simulink model "logical_hystersis_prove"  (R2014b)
settings: Solver=FixedStepDiscrete  StartTime=0.0  StopTime=0.03  FixedStep=0.01  RelTol=1e-3
undefined symbols (not defined in the file): sldvsubsys
libraries: sldvlib x16
settings Model: Creator=Natasha  LastModifiedBy=JYOGANAN
settings DebuggingCC: UnderspecifiedInitializationDetection=Classic  MergeDetectMultiDrivingBlocksExec=none

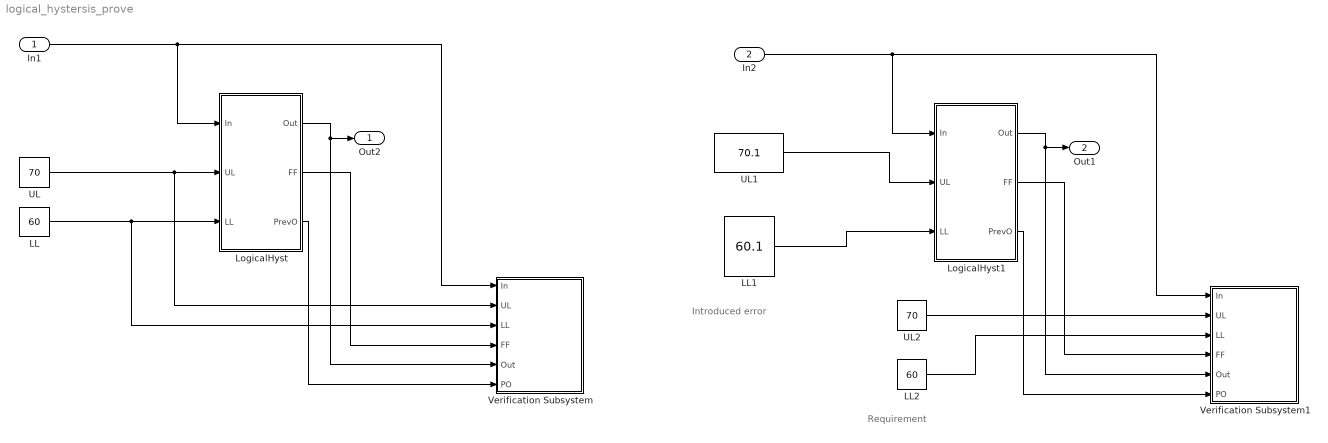
== system logical_hystersis_prove ==
  note: Introduced error
  note: Requirement
  In1 : Inport
  In2 : Inport  Port=2
  LL : Constant  Value=60
  LL1 : Constant  Value=60.1
  LL2 : Constant  Value=60
  LogicalHyst : Subsystem
  LogicalHyst1 : Subsystem
  UL : Constant  Value=70
  UL1 : Constant  Value=70.1
  UL2 : Constant  Value=70
  Verification Subsystem : Subsystem  Tag=VerificationSubsystem  DisableCoverage=on  LoadFcn=sldvsubsys('check')  TreatAsAtomicUnit=on  SimViewingDevice=on  mask(VerificationSubsystem){}
      mask init:
      | sldvsubsys('maskInit');
      settings: CopyFcn=sldvsubsys('copy');  OpenFcn=open_system(gcb,'force');
      settings: PreSaveFcn=|
      | set_param(gcb,'SimViewingDevice','on');
      | sldvsubsys('check');
      mask Help: helpview(fullfile(docroot,'toolbox','sldv','sldv.map'),'verificationsubsystem')
      mask Display: image(imread('sldvicon_versubsys.png','BackGroundColor',[1 1 1]),'center');
  Verification Subsystem1 : Subsystem  Tag=VerificationSubsystem  DisableCoverage=on  LoadFcn=sldvsubsys('check')  TreatAsAtomicUnit=on  SimViewingDevice=on  mask(VerificationSubsystem){}
      mask init:
      | sldvsubsys('maskInit');
      settings: CopyFcn=sldvsubsys('copy');  OpenFcn=open_system(gcb,'force');
      settings: PreSaveFcn=|
      | set_param(gcb,'SimViewingDevice','on');
      | sldvsubsys('check');
      mask Help: helpview(fullfile(docroot,'toolbox','sldv','sldv.map'),'verificationsubsystem')
      mask Display: image(imread('sldvicon_versubsys.png','BackGroundColor',[1 1 1]),'center');
  Out2 : Outport
  Out1 : Outport  Port=2
  wires:
  UL/1 -> Verification Subsystem/2(UL), LogicalHyst/2(UL)
  LL/1 -> Verification Subsystem/3(LL), LogicalHyst/3(LL)
  LogicalHyst/1(Out) -> Verification Subsystem/5(Out), Out2/1
  LogicalHyst/2(FF) -> Verification Subsystem/4(FF)
  In1/1 -> LogicalHyst/1(In), Verification Subsystem/1(In)
  LogicalHyst/3(PrevO) -> Verification Subsystem/6(PO)
  UL1/1 -> LogicalHyst1/2(UL)
  LL1/1 -> LogicalHyst1/3(LL)
  LogicalHyst1/1(Out) -> Verification Subsystem1/5(Out), Out1/1
  LogicalHyst1/2(FF) -> Verification Subsystem1/4(FF)
  In2/1 -> LogicalHyst1/1(In), Verification Subsystem1/1(In)
  LogicalHyst1/3(PrevO) -> Verification Subsystem1/6(PO)
  UL2/1 -> Verification Subsystem1/2(UL)
  LL2/1 -> Verification Subsystem1/3(LL)

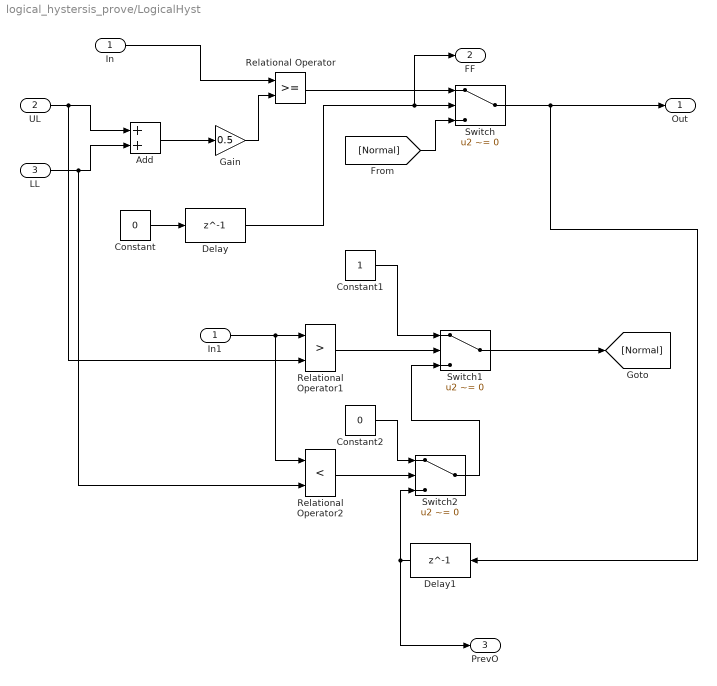
== system logical_hystersis_prove/LogicalHyst ==
  In : Inport
  UL : Inport  Port=2
  LL : Inport  Port=3
  Add : Sum
  Constant : Constant  Value=0
  Constant1 : Constant  OutDataTypeStr=boolean
  Constant2 : Constant  Value=0  OutDataTypeStr=boolean
  Delay : Delay  DelayLength=1  InitialCondition=1
  Delay1 : Delay  DelayLength=1  InitialCondition=0
  Gain : Gain  Gain=0.5
  In1 : InportShadow
  Relational Operator : RelationalOperator  OutDataTypeStr=boolean
  Relational Operator1 : RelationalOperator  Operator=>  OutDataTypeStr=boolean
  Relational Operator2 : RelationalOperator  Operator=<  OutDataTypeStr=boolean
  Switch : Switch  Criteria=u2 ~= 0
  Switch1 : Switch  Criteria=u2 ~= 0
  Switch2 : Switch  Criteria=u2 ~= 0
  Out : Outport
  FF : Outport  Port=2
  PrevO : Outport  Port=3
  wires:
  In/1 -> Relational Operator/1
  Constant/1 -> Delay/1
  Switch/1 -> Delay1/1, Out/1
  UL/1 -> Relational Operator1/2, Add/1
  Delay/1 -> FF/1, Switch/2
  [Normal] -> Switch/3
  Add/1 -> Gain/1
  LL/1 -> Relational Operator2/2, Add/2
  Gain/1 -> Relational Operator/2
  Relational Operator/1 -> Switch/1
  In1/1 -> Relational Operator2/1, Relational Operator1/1
  Relational Operator1/1 -> Switch1/2
  Constant1/1 -> Switch1/1
  Relational Operator2/1 -> Switch2/2
  Constant2/1 -> Switch2/1
  Switch2/1 -> Switch1/3
  Switch1/1 -> [Normal]
  Delay1/1 -> Switch2/3, PrevO/1

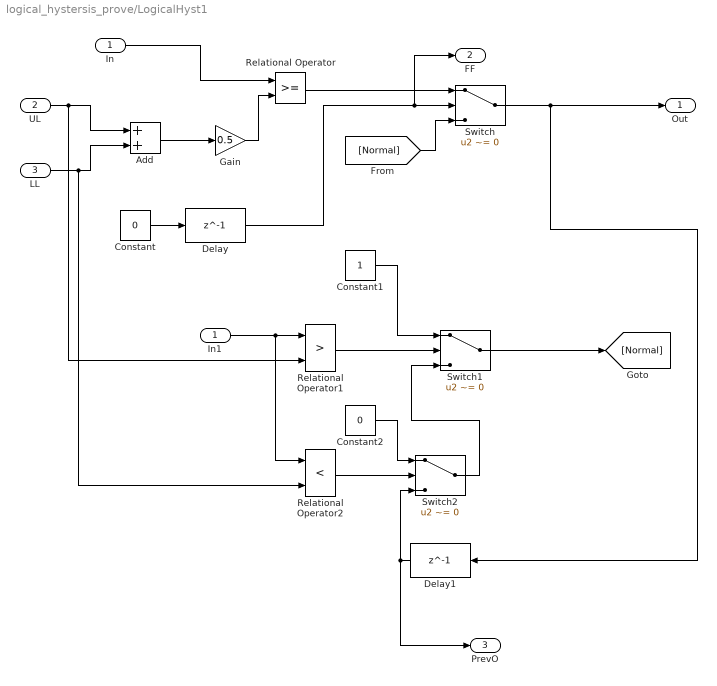
== system logical_hystersis_prove/LogicalHyst1 ==
  In : Inport
  UL : Inport  Port=2
  LL : Inport  Port=3
  Add : Sum
  Constant : Constant  Value=0
  Constant1 : Constant  OutDataTypeStr=boolean
  Constant2 : Constant  Value=0  OutDataTypeStr=boolean
  Delay : Delay  DelayLength=1  InitialCondition=1
  Delay1 : Delay  DelayLength=1  InitialCondition=0
  Gain : Gain  Gain=0.5
  In1 : InportShadow
  Relational Operator : RelationalOperator  OutDataTypeStr=boolean
  Relational Operator1 : RelationalOperator  Operator=>  OutDataTypeStr=boolean
  Relational Operator2 : RelationalOperator  Operator=<  OutDataTypeStr=boolean
  Switch : Switch  Criteria=u2 ~= 0
  Switch1 : Switch  Criteria=u2 ~= 0
  Switch2 : Switch  Criteria=u2 ~= 0
  Out : Outport
  FF : Outport  Port=2
  PrevO : Outport  Port=3
  wires:
  In/1 -> Relational Operator/1
  Constant/1 -> Delay/1
  Switch/1 -> Delay1/1, Out/1
  UL/1 -> Relational Operator1/2, Add/1
  Delay/1 -> FF/1, Switch/2
  [Normal] -> Switch/3
  Add/1 -> Gain/1
  LL/1 -> Relational Operator2/2, Add/2
  Gain/1 -> Relational Operator/2
  Relational Operator/1 -> Switch/1
  In1/1 -> Relational Operator2/1, Relational Operator1/1
  Relational Operator1/1 -> Switch1/2
  Constant1/1 -> Switch1/1
  Relational Operator2/1 -> Switch2/2
  Constant2/1 -> Switch2/1
  Switch2/1 -> Switch1/3
  Switch1/1 -> [Normal]
  Delay1/1 -> Switch2/3, PrevO/1

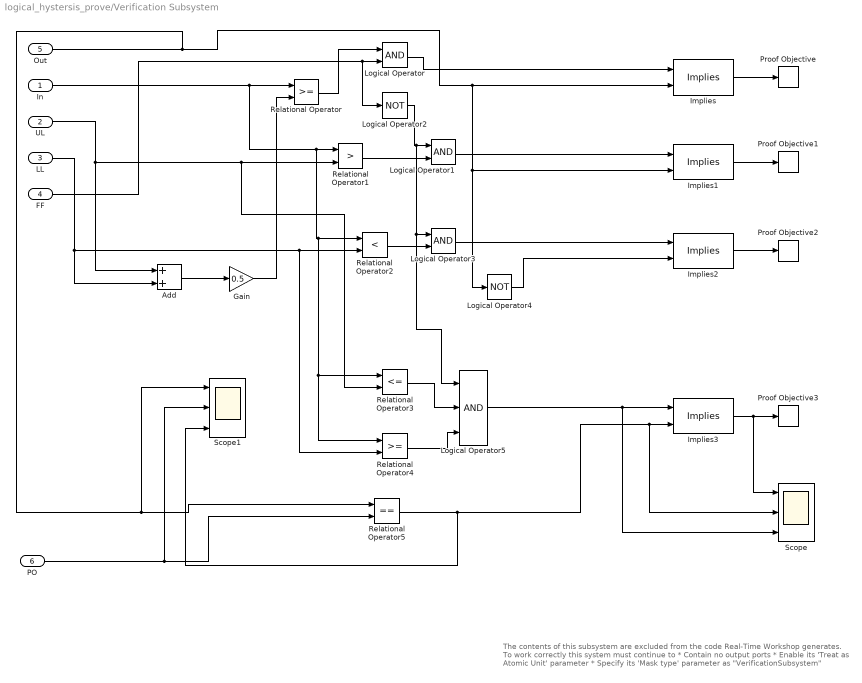
== system logical_hystersis_prove/Verification Subsystem ==
  note: The contents of this subsystem are excluded from the code Real-Time
      | Workshop generates.
      |
      | To work correctly this system must continue to
      | * Contain no output ports
      | * Enable its 'Treat as Atomic Unit' parameter
      | * Specify its 'Mask type' parameter as "VerificationSubsystem"
  In : Inport
  UL : Inport  Port=2
  LL : Inport  Port=3
  FF : Inport  Port=4
  Out : Inport  Port=5
  PO : Inport  Port=6
  Add : Sum
  Gain : Gain  Gain=0.5
  Implies{,1..3} (4 alike) : sldvlib/Verification Utilities/Implies
  Logical Operator : Logic  AllPortsSameDT=off  OutDataTypeStr=boolean
  Logical Operator1 : Logic  AllPortsSameDT=off  OutDataTypeStr=boolean
  Logical Operator2 : Logic  Operator=NOT  AllPortsSameDT=off  OutDataTypeStr=boolean
  Logical Operator3 : Logic  AllPortsSameDT=off  OutDataTypeStr=boolean
  Logical Operator4 : Logic  Operator=NOT  AllPortsSameDT=off  OutDataTypeStr=boolean
  Logical Operator5 : Logic  Inputs=3  AllPortsSameDT=off  OutDataTypeStr=boolean
  Proof Objective{,1..3} (4 alike) : sldvlib/Objectives and Constraints/Proof Objective  enabled=on  customAVTBlockType=Proof Objective  intervals=true  dispValues=on  outEnabled=off  enableStopSim=off
      settings: AttributesFormatString=%<intervals>
  Relational Operator : RelationalOperator  OutDataTypeStr=boolean
  Relational Operator1 : RelationalOperator  Operator=>  OutDataTypeStr=boolean
  Relational Operator2 : RelationalOperator  Operator=<  OutDataTypeStr=boolean
  Relational Operator3 : RelationalOperator  Operator=<=  OutDataTypeStr=boolean
  Relational Operator4 : RelationalOperator  OutDataTypeStr=boolean
  Relational Operator5 : RelationalOperator  Operator===  OutDataTypeStr=boolean
  Scope : Scope  NumInputPorts=3
      settings: YMin=-5~-5~-5  YMax=5~5~5
  Scope1 : Scope  NumInputPorts=3
      settings: YMin=-5~-5~-5  YMax=5~5~5
  wires:
  FF/1 -> Logical Operator2/1, Logical Operator/2
  Out/1 -> Scope1/1, Relational Operator5/1, Logical Operator4/1, Implies1/2, Implies/2
  Logical Operator/1 -> Implies/1
  Relational Operator/1 -> Logical Operator/1
  In/1 -> Relational Operator3/1, Relational Operator4/1, Relational Operator2/1, Relational Operator1/1, Relational Operator/1
  Add/1 -> Gain/1
  UL/1 -> Relational Operator3/2, Relational Operator1/2, Add/1
  LL/1 -> Relational Operator4/2, Relational Operator2/2, Add/2
  Gain/1 -> Relational Operator/2
  Relational Operator1/1 -> Logical Operator1/2
  Logical Operator2/1 -> Logical Operator5/1, Logical Operator3/1, Logical Operator1/1
  Logical Operator1/1 -> Implies1/1
  Logical Operator3/1 -> Implies2/1
  Relational Operator2/1 -> Logical Operator3/2
  Logical Operator4/1 -> Implies2/2
  Relational Operator3/1 -> Logical Operator5/2
  Relational Operator4/1 -> Logical Operator5/3
  Logical Operator5/1 -> Scope/3, Implies3/1
  Relational Operator5/1 -> Scope1/3, Scope/2, Implies3/2
  Implies/1 -> Proof Objective/1
  Implies1/1 -> Proof Objective1/1
  Implies2/1 -> Proof Objective2/1
  Implies3/1 -> Scope/1, Proof Objective3/1
  PO/1 -> Scope1/2, Relational Operator5/2

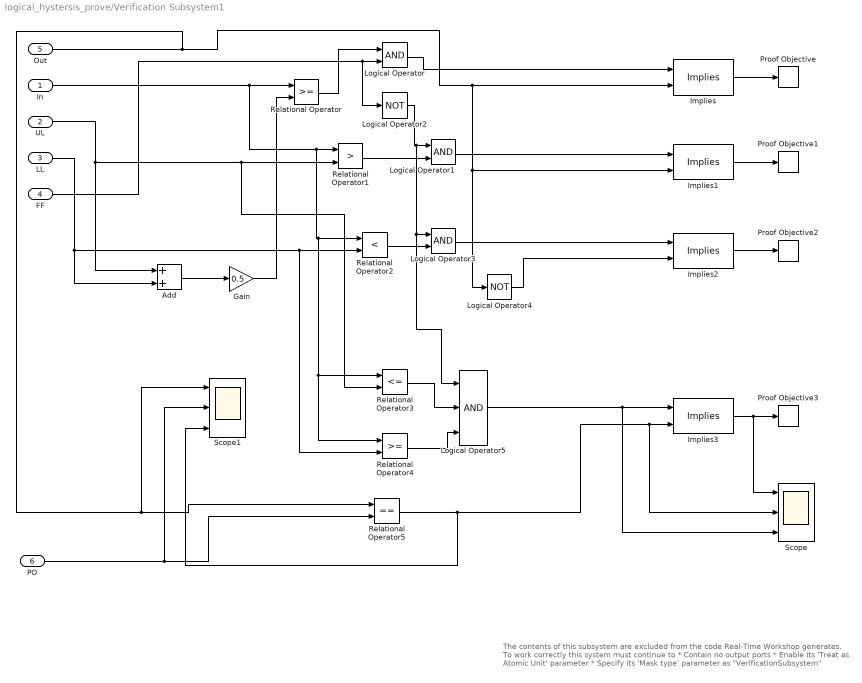
== system logical_hystersis_prove/Verification Subsystem1 ==
  note: The contents of this subsystem are excluded from the code Real-Time
      | Workshop generates.
      |
      | To work correctly this system must continue to
      | * Contain no output ports
      | * Enable its 'Treat as Atomic Unit' parameter
      | * Specify its 'Mask type' parameter as "VerificationSubsystem"
  In : Inport
  UL : Inport  Port=2
  LL : Inport  Port=3
  FF : Inport  Port=4
  Out : Inport  Port=5
  PO : Inport  Port=6
  Add : Sum
  Gain : Gain  Gain=0.5
  Implies{,1..3} (4 alike) : sldvlib/Verification Utilities/Implies
  Logical Operator : Logic  AllPortsSameDT=off  OutDataTypeStr=boolean
  Logical Operator1 : Logic  AllPortsSameDT=off  OutDataTypeStr=boolean
  Logical Operator2 : Logic  Operator=NOT  AllPortsSameDT=off  OutDataTypeStr=boolean
  Logical Operator3 : Logic  AllPortsSameDT=off  OutDataTypeStr=boolean
  Logical Operator4 : Logic  Operator=NOT  AllPortsSameDT=off  OutDataTypeStr=boolean
  Logical Operator5 : Logic  Inputs=3  AllPortsSameDT=off  OutDataTypeStr=boolean
  Proof Objective{,1..3} (4 alike) : sldvlib/Objectives and Constraints/Proof Objective  enabled=on  customAVTBlockType=Proof Objective  intervals=true  dispValues=on  outEnabled=off  enableStopSim=off
      settings: AttributesFormatString=%<intervals>
  Relational Operator : RelationalOperator  OutDataTypeStr=boolean
  Relational Operator1 : RelationalOperator  Operator=>  OutDataTypeStr=boolean
  Relational Operator2 : RelationalOperator  Operator=<  OutDataTypeStr=boolean
  Relational Operator3 : RelationalOperator  Operator=<=  OutDataTypeStr=boolean
  Relational Operator4 : RelationalOperator  OutDataTypeStr=boolean
  Relational Operator5 : RelationalOperator  Operator===  OutDataTypeStr=boolean
  Scope : Scope  NumInputPorts=3
      settings: YMin=-5~-5~-5  YMax=5~5~5
  Scope1 : Scope  NumInputPorts=3
      settings: YMin=-5~-5~-5  YMax=5~5~5
  wires:
  FF/1 -> Logical Operator2/1, Logical Operator/2
  Out/1 -> Scope1/1, Relational Operator5/1, Logical Operator4/1, Implies1/2, Implies/2
  Logical Operator/1 -> Implies/1
  Relational Operator/1 -> Logical Operator/1
  In/1 -> Relational Operator3/1, Relational Operator4/1, Relational Operator2/1, Relational Operator1/1, Relational Operator/1
  Add/1 -> Gain/1
  UL/1 -> Relational Operator3/2, Relational Operator1/2, Add/1
  LL/1 -> Relational Operator4/2, Relational Operator2/2, Add/2
  Gain/1 -> Relational Operator/2
  Relational Operator1/1 -> Logical Operator1/2
  Logical Operator2/1 -> Logical Operator5/1, Logical Operator3/1, Logical Operator1/1
  Logical Operator1/1 -> Implies1/1
  Logical Operator3/1 -> Implies2/1
  Relational Operator2/1 -> Logical Operator3/2
  Logical Operator4/1 -> Implies2/2
  Relational Operator3/1 -> Logical Operator5/2
  Relational Operator4/1 -> Logical Operator5/3
  Logical Operator5/1 -> Scope/3, Implies3/1
  Relational Operator5/1 -> Scope1/3, Scope/2, Implies3/2
  Implies/1 -> Proof Objective/1
  Implies1/1 -> Proof Objective1/1
  Implies2/1 -> Proof Objective2/1
  Implies3/1 -> Scope/1, Proof Objective3/1
  PO/1 -> Scope1/2, Relational Operator5/2
